simulink model "speed_measurement"  (R2021b)
settings: Solver=FixedStepAuto  StartTime=0.0  StopTime=1  FixedStep=1e-6  RelTol=1e-3
libraries: fl_lib x8, nesl_utility x7, spsEdgeDetectorLib x3, ee_lib x2, eeGeneralControl x1
settings Model: Creator=adria  LastModifiedBy=adria

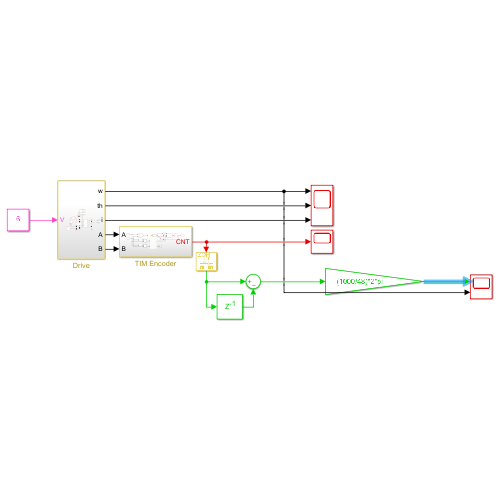
[thumbnail: Simulink's stored preview of the top-level diagram]
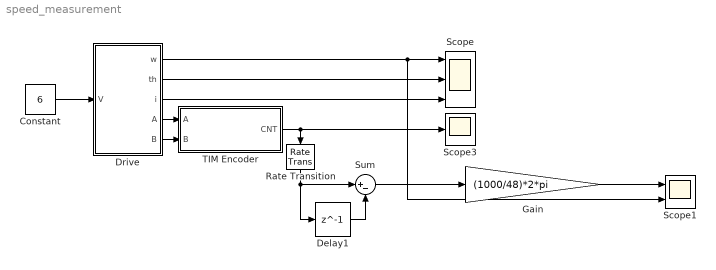
== system speed_measurement ==
  Constant : Constant  Value=6
  Delay1 : Delay  DelayLength=1  SampleTime=0.001
  Drive : Subsystem
  Gain : Gain  Gain=(1000/48)*2*pi
  Rate Transition : RateTransition  OutPortSampleTime=0.001
  Scope : Scope  NumInputPorts=3
  Scope1 : Scope  NumInputPorts=2
  Scope3 : Scope
  Sum : Sum  Inputs=|+-
  TIM Encoder : Subsystem
  wires:
  Constant/1 -> Drive/1(V)
  Drive/1(w) -> Scope/1, Scope1/2
  Drive/2(th) -> Scope/2
  Drive/3(i) -> Scope/3
  Drive/4(A) -> TIM Encoder/1(A)
  Drive/5(B) -> TIM Encoder/2(B)
  TIM Encoder/1(CNT) -> Rate Transition/1, Scope3/1
  Sum/1 -> Gain/1
  Gain/1 -> Scope1/1
  Rate Transition/1 -> Delay1/1, Sum/1
  Delay1/1 -> Sum/2

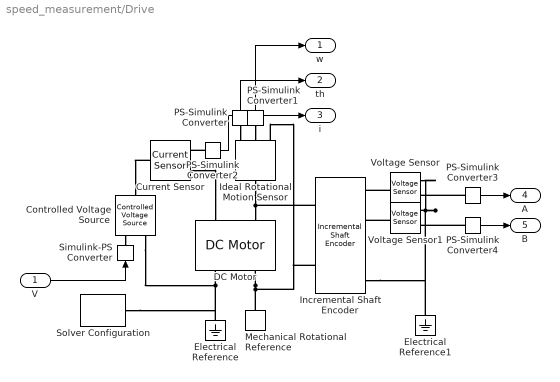
== system speed_measurement/Drive ==
  V : Inport
  Controlled Voltage Source : fl_lib/Electrical/Electrical Sources/Controlled Voltage Source
  Current Sensor : fl_lib/Electrical/Electrical Sensors/Current Sensor
  DC Motor : ee_lib/Electromechanical/Brushed Motors/DC Motor  field_option=ee.enum.field_option.pm  Rf=100 Ohm  Lf=1 H  Laf=0.15 H  If0=0 A  parameterization=ee.enum.dcparam_option.circuit_param  Ra=4e+0 Ohm  La=1e-4 H  emf_or_torque=ee.enum.emf_or_torque.kv  Kv=2e-3 V/(rad/s)  Ki=6.876e-4 N*m/A  T_stall=0.24e-3 N*m  w_max=19100 rpm  w_rated=15000 rpm  P_rated=0.08 W  V_rated=1.5 V  lam_param=ee.enum.lam_param.damping  i_noload=0 A  V_i_noload=1.5 V  J=1e-7 kg*m^2  lam=0 N*m/(rad/s)  speed0=0 rpm  enable_fault_armature=simscape.enum.onoff.off  rev_faulted=1 / 3  G_faulted_armature=1e-5 S  fault_trigger_armature=ee.enum.faults.faultTrigger.temporal  t_fault_armature=1 s  max_permissible_current_armature=inf A  t_fail_on_current_armature=1 s  enable_fault_field=simscape.enum.onoff.off  G_faulted_field=1e-5 S  fault_trigger_field=ee.enum.faults.faultTrigger.temporal  t_fault_field=1 s  max_permissible_current_field=inf A  t_fail_on_current_field=1 s  fault_action=simscape.enum.assert.action.none  alpha=3.93e-3 1/K  Tmeas=25 degC  thermal_mass=100 J/K  initial_temperature=25 degC
  Electrical Reference : fl_lib/Electrical/Electrical Elements/Electrical Reference
  Electrical Reference1 : fl_lib/Electrical/Electrical Elements/Electrical Reference
  Ideal Rotational Motion Sensor : fl_lib/Mechanical/Mechanical Sensors/Ideal Rotational Motion Sensor  wrap_angle=simscape.enum.onoff.on  offset=0 rad
  Incremental Shaft Encoder : ee_lib/Sensors & Transducers/Incremental Shaft Encoder  NPulse=12  Vm=3.3 V  angle0=0 deg
      settings: SourceProductBaseCode=PS  InternalSimscapePortConfiguration="{\"Bottom\":[],\"Left\":[{\"id\":\"R\",\"label\":\"R\",\"type\":\"foundation.mechanical.rotational.rotational\"},{\"id\":\"C\",\"label\":\"C\",\"type\":\"foundation.mechanical.rotational.rotational\"}],\"Right\":[{\"id\":\"A\",\"label\":\"A\",\"type\":\"foundation.electrical.electrical\"},{\"id\":\"B\",\"label\":\"B\",\"type\":\"foundation.electrical.electrical\"},{\"id\":\"Z\",\"label\":\"Z\",\"type\":\"foundation.electrical.electrical\"},{\"id\":\"GND\",\"label\":\"REF\",\"type\":\"foundation.electrical.electrical\"}],\"Top\":[]}"
  Mechanical Rotational Reference : fl_lib/Mechanical/Rotational Elements/Mechanical Rotational Reference
  PS-Simulink Converter{,1..4} (5 alike) : nesl_utility/PS-Simulink Converter  PhysicalDomain=network_engine_domain  SubClassName=ps_output  LeftPortType=input  RightPortType=output  PseudoPeriodic=off  Frequencies=[]  Unit=inherit  AffineConversion=off
      settings: SourceProductBaseCode=PW,SS
  Simulink-PS Converter : nesl_utility/Simulink-PS Converter  PhysicalDomain=network_engine_domain  SubClassName=ps_input  LeftPortType=input  RightPortType=output  PseudoPeriodic=off  Frequencies=[]  NoiseDistribution=none  NoiseParameters=[]  Unit=1  AffineConversion=off  FilteringAndDerivatives=provide  SimscapeFilterOrder=1  InputFilterTimeConstant=0.001  UdotUserProvided=0
      settings: SourceProductBaseCode=PW,SS
  Solver Configuration : nesl_utility/Solver Configuration  PhysicalDomain=network_engine_domain  SubClassName=solver  LeftPortType=input  RightPortType=generic  Tones=[]  Harmonics=[]  SimulateNoise=off  Profile=off  UseLocalSampling=off  EnableSwitchedLinearOptims=on  FrequencyDomain=off  UseCCode=off  RelTol=0.001  AbsTol=1e-06  MinStep=1e-09  ToWorkspace=off  RevertToSquareIcSolve=off  NumHomotopyIterations=100  PhasorMode=off  PhasorModeNumHarmonics=1  DoDC=off  ResidualTolerance=1e-09  UseLocalSolver=off  LocalSolverChoice=NE_BACKWARD_EULER_ADVANCER  LocalSolverSampleTime=0.001  DoFixedCost=off  MaxNonlinIter=3  MaxModeIter=2  ComputeImpulses=off  ImpulseIterations=2  LinearAlgebra=auto  EquationFormulation=NE_TIME_EF  DelaysMemoryBudget=1024  AutomaticFiltering=on  FilteringTimeConstant=0.001  PartitionStorageMethod=AS_NEEDED  PartitionMemoryBudget=1024  PartitionMethod=ROBUST
      settings: SourceProductBaseCode=PW,SS
  Voltage Sensor : fl_lib/Electrical/Electrical Sensors/Voltage Sensor
  Voltage Sensor1 : fl_lib/Electrical/Electrical Sensors/Voltage Sensor
  w : Outport
  th : Outport  Port=2
  i : Outport  Port=3
  A : Outport  Port=4
  B : Outport  Port=5
  wires:
  PS-Simulink Converter2/1 -> i/1
  PS-Simulink Converter/1 -> th/1
  PS-Simulink Converter3/1 -> A/1
  V/1 -> Simulink-PS Converter/1
  PS-Simulink Converter4/1 -> B/1
  PS-Simulink Converter1/1 -> w/1
  connections:
  DC Motor/RConn2 -- Ideal Rotational Motion Sensor/RConn1 -- Incremental Shaft Encoder/LConn2 -- Mechanical Rotational Reference/LConn1
  DC Motor/RConn1 -- Controlled Voltage Source/RConn2 -- Electrical Reference/LConn1 -- Solver Configuration/RConn1
  Voltage Sensor1/RConn2 -- Electrical Reference1/LConn1 -- Incremental Shaft Encoder/RConn4 -- Voltage Sensor/RConn2
  Incremental Shaft Encoder/LConn1 -- Ideal Rotational Motion Sensor/LConn1 -- DC Motor/LConn2
  Voltage Sensor/LConn1 -- Incremental Shaft Encoder/RConn1
  PS-Simulink Converter3/LConn1 -- Voltage Sensor/RConn1
  Voltage Sensor1/LConn1 -- Incremental Shaft Encoder/RConn2
  Current Sensor/LConn1 -- Controlled Voltage Source/LConn1
  PS-Simulink Converter1/LConn1 -- Ideal Rotational Motion Sensor/RConn2
  PS-Simulink Converter/LConn1 -- Ideal Rotational Motion Sensor/RConn3
  Controlled Voltage Source/RConn1 -- Simulink-PS Converter/RConn1
  PS-Simulink Converter2/LConn1 -- Current Sensor/RConn1
  PS-Simulink Converter4/LConn1 -- Voltage Sensor1/RConn1
  Current Sensor/RConn2 -- DC Motor/LConn1

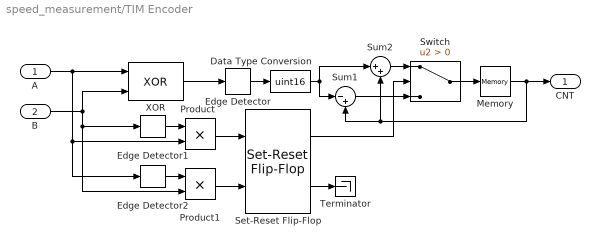
== system speed_measurement/TIM Encoder ==
  A : Inport
  B : Inport  Port=2
  Data Type Conversion : DataTypeConversion  OutDataTypeStr=uint16
  Edge Detector : spsEdgeDetectorLib/Edge Detector  model=Either  ic=0  Ts=0
      settings: SourceProductBaseCode=PS
  Edge Detector1 : spsEdgeDetectorLib/Edge Detector  model=Rising  ic=0  Ts=0
      settings: SourceProductBaseCode=PS
  Edge Detector2 : spsEdgeDetectorLib/Edge Detector  model=Rising  ic=0  Ts=0
      settings: SourceProductBaseCode=PS
  Memory : Memory
  Product : Product
  Product1 : Product
  Set-Reset Flip-Flop : eeGeneralControl/Set-Reset Flip-Flop  LabelModeActiveChoice=Discrete  UndefState=Set  Q0=1  Ts=-1
      settings: SourceProductBaseCode=PS
  Sum1 : Sum  Inputs=|-+
  Sum2 : Sum  Inputs=|++
  Switch : Switch  Criteria=u2 > Threshold
  Terminator : Terminator
  XOR : Logic  Operator=XOR  IconShape=distinctive  AllPortsSameDT=off  OutDataTypeStr=boolean
  CNT : Outport
  wires:
  Set-Reset Flip-Flop/2 -> Terminator/1
  Product/1 -> Set-Reset Flip-Flop/1
  Data Type Conversion/1 -> Sum1/1, Sum2/1
  Product1/1 -> Set-Reset Flip-Flop/2
  Set-Reset Flip-Flop/1 -> Switch/2
  Edge Detector/1 -> Data Type Conversion/1
  B/1 -> XOR/2, Product1/2, Edge Detector1/1
  XOR/1 -> Edge Detector/1
  Switch/1 -> Memory/1
  A/1 -> Edge Detector2/1, Product/2, XOR/1
  Edge Detector1/1 -> Product/1
  Sum2/1 -> Switch/1
  Memory/1 -> CNT/1, Sum2/2, Sum1/2
  Edge Detector2/1 -> Product1/1
  Sum1/1 -> Switch/3
